simulink model "test"  (R2025a)
settings: Solver=FixedStepAuto  StartTime=0.0  StopTime=inf  FixedStep=0.0201  RelTol=1e-3  EnableMultiTasking=on
InitFcn:
  | load2slx
model workspace (MAT data in the model file):
  F = [1.0101  0  0; 0  1.0101  0; 0  0  1.0101; 1.02030201  0  0; 0  1.02030201  0; 0  0  1.02030201; 1.0306070603  0  0; 0  1.0306070603  0; 0  0  1.0306070603; 1.04101619161  0  0; 0  1.04101619161  0; 0  0  1.04101619161; 1.05153045515  0  0; 0  1.05153045515  0; 0  0  1.05153045515]
  G = [0.3357  0  0  0  0  0  0  0  0  0  0  0  0  0  0; 0  0.9698  0  0  0  0  0  0  0  0  0  0  0  0  0; 0  0  0.0305  0  0  0  0  0  0  0  0  0  0  0  0; 0.33909057  0  0  0.3357  0  0  0  0  0  0  0  0  0  0  0; 0  0.97959498  0  0  0.9698  0  0  0  0  0  0  0  0  0  0; 0  0  0.03080805  0  0  0.0305  0  0  0  0  0  0  0  0  0; 0.342515384757  0  0  0.33909057  0  0  0.3357  0  0  0  0  0  0  0  0; 0  0.989488889298  0  0  0.97959498  0  0  0.9698  0  0  0  0  0  0  0; 0  0  0.031119211305  0  0  0.03080805  0  0  0.0305  0  0  0  0  0  0; 0.345974790143  0  0  0.342515384757  0  0  0.33909057  0  0  0.3357  0  0  0  0  0; 0  0.99948272708  0  0  0.989488889298  0  0  0.97959498  0  0  0.9698  0  0  0  0; 0  0  0.0314335153392  0  0  0.031119211305  0  0  0.03080805  0  0  0.0305  0  0  0; 0.349469135523  0  0  0.345974790143  0  0  0.342515384757  0  0  0.33909057  0  0  0.3357  0  0; 0  1.00957750262  0  0  0.99948272708  0  0  0.989488889298  0  0  0.97959498  0  0  0.9698  0; 0  0  0.0317509938441  0  0  0.0314335153392  0  0  0.031119211305  0  0  0.03080805  0  0  0.0305]
  H = [1.90762936235 -3.65415117825e-17 0 0.786986310617 -3.61761328408e-17 0 0.666422736628 -3.58144073268e-17 0 0.545926464672 -3.54562987099e-17 0 ... (225 elements, 15x15)]
  Pc = [-0.3357 0 0 0.3357 0 0 -0.33909057 0 0 0.33909057 0 0 ... (990 elements, 66x15)]
  Qvec = [1  0  0  0  0  0  0  0  0  0  0  0  0  0  0; 0  1  0  0  0  0  0  0  0  0  0  0  0  0  0; 0  0  1  0  0  0  0  0  0  0  0  0  0  0  0; 0  0  0  1  0  0  0  0  0  0  0  0  0  0  0; 0  0  0  0  1  0  0  0  0  0  0  0  0  0  0; 0  0  0  0  0  1  0  0  0  0  0  0  0  0  0; 0  0  0  0  0  0  1  0  0  0  0  0  0  0  0; 0  0  0  0  0  0  0  1  0  0  0  0  0  0  0; 0  0  0  0  0  0  0  0  1  0  0  0  0  0  0; 0  0  0  0  0  0  0  0  0  1  0  0  0  0  0; 0  0  0  0  0  0  0  0  0  0  1  0  0  0  0; 0  0  0  0  0  0  0  0  0  0  0  1  0  0  0; 0  0  0  0  0  0  0  0  0  0  0  0  3.62680678699  -1.03570964587e-16  0; 0  0  0  0  0  0  0  0  0  0  0  0  -1.03570964587e-16  1.66151464552  0; 0  0  0  0  0  0  0  0  0  0  0  0  0  0  46.1283533727]
  Sc = [1.0101  0  0; 0  1.0101  0; 0  0  1.0101; -1.0101  0  0; 0  -1.0101  0; 0  0  -1.0101; 1.02030201  0  0; 0  1.02030201  0; 0  0  1.02030201; -1.02030201  0  0; 0  -1.02030201  0; 0  0  -1.02030201; 1.0306070603  0  0; 0  1.0306070603  0; 0  0  1.0306070603; -1.0306070603  0  0; 0  -1.0306070603  0; 0  0  -1.0306070603; 1.04101619161  0  0; 0  1.04101619161  0; 0  0  1.04101619161; -1.04101619161  0  0; 0  -1.04101619161  0; 0  0  -1.04101619161; 1.05153045515  0  0; 0  1.05153045515  0; 0  0  1.05153045515; -1.05153045515  0  0; 0  -1.05153045515  0; 0  0  -1.05153045515; 0  0  0; 0  0  0; 0  0  0; 0  0  0; 0  0  0; 0  0  0; 0  0  0; 0  0  0; 0  0  0; 0  0  0; 0  0  0; 0  0  0; 0  0  0; 0  0  0; 0  0  0; 0  0  0; 0  0  0; 0  0  0; 0  0  0; 0  0  0; 0  0  0; 0  0  0; 0  0  0; 0  0  0; 0  0  0; 0  0  0; 0  0  0; 0  0  0; 0  0  0; 0  0  0; 1.05153045515  0  0; 0  1.05153045515  0; 0  0  1.05153045515; -1.05153045515  0  0; 0  -1.05153045515  0; 0  0  -1.05153045515]
  m = 3
  nu = 15
  qc = [1; 1; 0.5; 1; 1; 0.5; 1; 1; 0.5; 1; 1; 0.5; 1; 1; 0.5; 1; 1; 0.5; 1; 1; 0.5; 1; 1; 0.5; 1; 1; 0.5; 1; 1; 0.5; 1.41421356237; 1.41421356237; 2; 1.41421356237; 1.41421356237; 2; 1.41421356237; 1.41421356237; 2; 1.41421356237; 1.41421356237; 2; 1.41421356237; 1.41421356237; 2; 1.41421356237; 1.41421356237; 2; 1.41421356237; 1.41421356237; 2; 1.41421356237; 1.41421356237; 2; 1.41421356237; 1.41421356237; 2; 1.41421356237; 1.41421356237; 2; 1; 1; 0.5; 1; 1; 0.5]
settings Model: SimulationMode=external  ExtModeTrigDuration=10  Creator=The MathWorks, Inc.  LastModifiedBy=aero
settings SolverCC: AlgebraicLoopSolver=TrustRegion  PositivePriorityOrder=on  AutoInsertRateTranBlk=on  MaxZcPerStep=1.0
settings OptimizationCC: EnhancedBackFolding=on  PassReuseOutputArgsAs=Individual arguments  MaxStackSize=64  OptimizeBlockOrder=speed  DifferentSizesBufferReuse=on  OptimizationCustomize=off  EfficientTunableParamExpr=on
settings DebuggingCC: ParameterPrecisionLossMsg=none  ParameterTunabilityLossMsg=error  UnconnectedInputMsg=warning  UnconnectedOutputMsg=warning  UnconnectedLineMsg=warning  SubsystemReferenceDiagnosticForUnitTest=warning  ArithmeticOperatorsInVariantConditions=warning
settings HardwareCC: ProdBitPerPointer=32.0  ProdBitPerSizeT=32.0  ProdBitPerPtrDiffT=32.0  ProdLargestAtomicInteger=Long  ProdLargestAtomicFloat=Double  ProdWordSize=32.0  ProdLongLongMode=on  ProdHWDeviceType=ARM Compatible->ARM Cortex
settings ModelReferenceCC: EnableRefExpFcnMdlSchedulingChecks=on
settings SFSimCC: MATLABDynamicMemAlloc=off  SimTargetLang=C++  SimDLTargetLibrary=mkl-dnn
settings RTWCC: SystemTargetFile=ert.tlc  HardwareBoard=PX4 Pixhawk 6c  TLCOptions="-aInlineSetEventsForThisBaseRateFcn=TLC_FALSE -aSuppressMultiTaskScheduler=TLC_FALSE  -aRateBasedStepFcn=0"  TemplateMakefile=ert_default_tmf  GenerateReport=on  Toolchain=GNU Tools for PX4 Autopilots  IncludeHyperlinkInReport=on  LaunchReport=on  TargetLang=C++  GenerateTraceInfo=on  GenerateTraceReport=on  GenerateTraceReportSl=on  GenerateTraceReportSf=on  GenerateTraceReportEml=on  GPUComputeCapability=3.5  DLArmComputeVersion=19.05  Description=Embedded Coder
settings CodeAppCC: ForceParamTrailComments=on  IgnoreCustomStorageClasses=off  OperatorAnnotations=on  SimulinkDataObjDesc=on  SFDataObjDesc=on  InsertBlockDesc=on
settings ERTTargetCC: ExtModeTransport=3.0  ExtModeStaticAllocSize=1024.0  InlinedParameterPlacement=Hierarchical

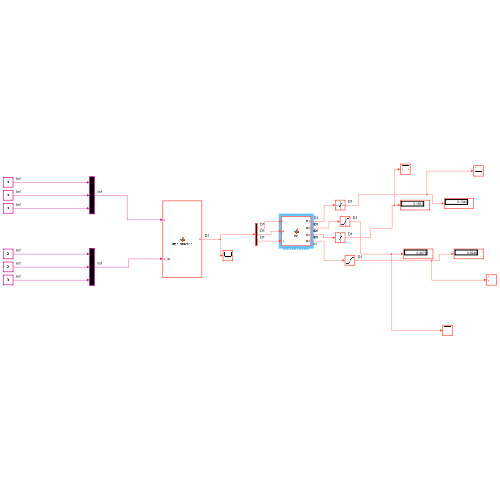
[thumbnail: Simulink's stored preview of the top-level diagram]
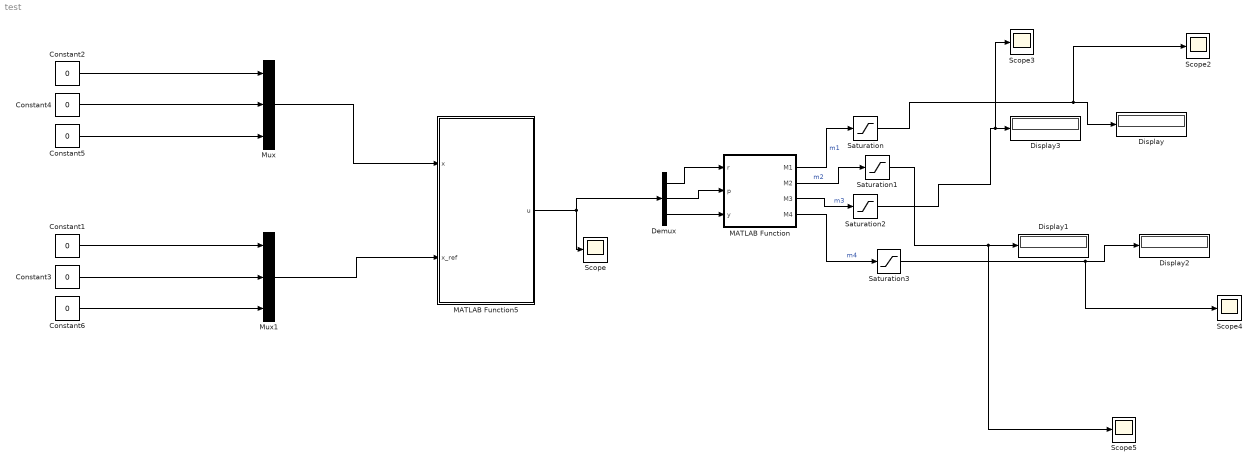
== system test ==
  Constant{1..6} (6 alike) : Constant  Value=0
  Demux : Demux  Outputs=3
  Display{,1..3} (4 alike) : Display
  MATLAB Function : MATLAB Function  TreatAsAtomicUnit=on  SystemSampleTime=0.0201
  MATLAB Function5 : MATLAB Function  TreatAsAtomicUnit=on  SystemSampleTime=0.0201
  Mux : Mux  Inputs=3
  Mux1 : Mux  Inputs=3
  Saturation{,1..3} (4 alike) : Saturate  UpperLimit=1  LowerLimit=0
  Scope{,2..5} (5 alike) : Scope
      Scope settings: ActiveDisplayYMinimum=-0.053985449326909025  ActiveDisplayYMaximum=0.097577906132606917
      Scope2 settings: DataLoggingVariableName=ScopeData2
      Scope3 settings: DataLoggingVariableName=ScopeData3
      Scope4 settings: DataLoggingVariableName=ScopeData4
      Scope5 settings: DataLoggingVariableName=ScopeData5
  wires:
  MATLAB Function/2(M2) -> Saturation1/1  "m2"
  Demux/3 -> MATLAB Function/3(y)
  Demux/1 -> MATLAB Function/1(r)
  MATLAB Function5/1(u) -> Demux/1, Scope/1
  MATLAB Function/1(M1) -> Saturation/1  "m1"
  MATLAB Function/4(M4) -> Saturation3/1  "m4"
  Demux/2 -> MATLAB Function/2(p)
  MATLAB Function/3(M3) -> Saturation2/1  "m3"
  Saturation/1 -> Scope2/1, Display/1
  Saturation1/1 -> Scope5/1, Display1/1
  Saturation2/1 -> Scope3/1, Display3/1
  Mux/1 -> MATLAB Function5/1(x)
  Constant4/1 -> Mux/2
  Constant2/1 -> Mux/1
  Saturation3/1 -> Scope4/1, Display2/1
  Constant3/1 -> Mux1/2
  Constant1/1 -> Mux1/1
  Mux1/1 -> MATLAB Function5/2(x_ref)
  Constant5/1 -> Mux/3
  Constant6/1 -> Mux1/3

== matlab function test/MATLAB Function ==
  data: M1 output; r input; p input; y input; M2 output; M3 output; M4 output
function [M1,M2,M3,M4] = fcn( r, p, y)
% t: thrust
% r: roll
% p: pitch
% y: yaw
persistent trim mixer thrust
% M1 = t + r + p - y;
% M2 = t - r - p - y;
% M3 = t - r + p + y;
% M4 = t + r - p + y;
trim = [0.1344;0.2078;0.1551;0.2548];
thrust = 0;
u = [r;p;y; thrust];
mixer = [-1 1 1 -1;
        1 -1 1 -1;
        -1 -1 1 1
        1 1 1 1];
M = mixer\u;
M1= M(1,1)+trim(1,1);
M2= M(2,1)+trim(2,1);
M3= M(3,1)+trim(3,1);
M4= M(4,1)+trim(4,1);

== matlab function test/MATLAB Function5 ==
  data: x input; x_ref input; u output size=[m 1]; H parameter double; F parameter double; Qvec parameter double; G parameter double; Pc parameter double; qc parameter double; Sc parameter double
function u = mpc_function(x,x_ref, H, F, Qvec, G, Pc, qc, Sc)
persistent opts x0 u_prev
x = double(x);
x_ref= double(x_ref);
if isempty(u_prev)
    u_prev = zeros(3,1,'double');
end

if isempty(x0)
    x0 = zeros(15,1,'double');
end
x_tilde = x - x_ref;
% uvec = zeros(nu,1);

% === Construcción del QP ===
f = (2*x_tilde'*F'*Qvec*G)';

% Resolver QP
if isempty(opts)
opts = optimoptions('quadprog', 'Algorithm','active-set','Display','off');
end
[uvec,a,b] = quadprog(2*H,f, Pc,qc + Sc*x,[],[],[],[],x0, opts);

% Acción de control 
u = zeros(3,1);
if  b > 0
uvec = double(uvec);
u(:) = uvec(1:3);
u_prev = u;
x0= uvec;
else
    u = u_prev;
end
